simulink model "starmac_system"  (Simulink 7.1)
settings: Solver=ode5  StartTime=0.0  StopTime=30  FixedStep=.01  MaxStep=.01  RelTol=1e-4
undefined symbols (not defined in the file): ToverTh
libraries: xpcutilitieslib x19, simulink x10, xpclib x5, aero_sim_lib x1
settings Model: Creator=Administrator  LastModifiedBy=jporter  BufferReuse=off
settings OptimizationCC: BlockReduction=off  OptimizeBlockIOStorage=off  BufferReuse=off  ExpressionFolding=off  LocalBlockOutputs=off
settings HardwareCC: ProdIntDivRoundTo=Zero  ProdEndianess=LittleEndian  ProdHWDeviceType=Generic->32-bit x86 compatible
settings RTWCC: SystemTargetFile=xpctarget.tlc  TemplateMakefile=xpc_default_tmf  Description=xPC Target  ProcessScript=xpctarget_make_rtw_hook
settings xpcTargetCC: TargetFcnLib=ansi_tfl_table_tmw.mat  TargetFunctionLibrary=ANSI_C  CompOptLevelCompliant=off  PortableWordSizes=off  xPCisDownloadable=off

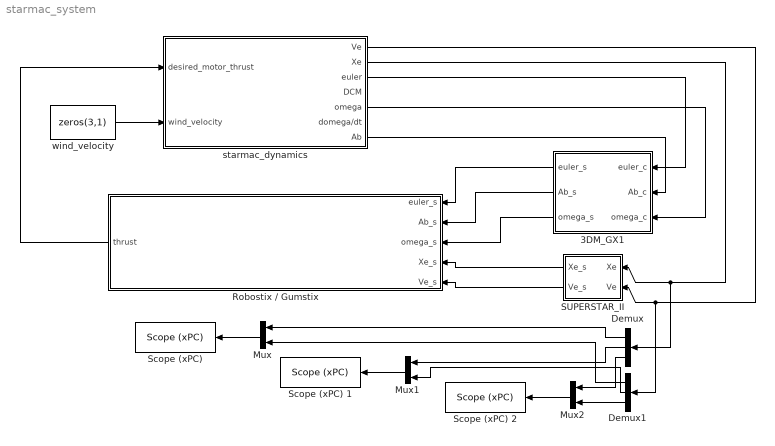
== system starmac_system ==
  3DM_GX1 : Subsystem  Orientation=left  mask{a_g_s=7000, g_max=5, g_g_s=8500, omega_max=300, Ts=.01}
      mask prompts: a_g_s "AccelGainScale:"; g_max "Max G (1 G = 9.81 m/s^2):"; g_g_s "GyroGainScale:"; omega_max "Mav Angular Velocity (deg/sec):"; Ts "Sample Rate (seconds):"
  Demux : Demux  Orientation=left  Outputs=3
  Demux1 : Demux  Orientation=left  Outputs=3
  Mux : Mux  Orientation=left  Inputs=2
  Mux1 : Mux  Orientation=left  Inputs=2
  Mux2 : Mux  Orientation=left  Inputs=2
  Robostix / Gumstix : Subsystem  Orientation=left
  SUPERSTAR_II : Subsystem  Orientation=left  mask{Ts=.2}
      mask prompts: Ts "Sample Rate (seconds):"
  "Scope (xPC) " : xpclib/Misc./Scope (xPC)   Orientation=left  SystemSampleTime=-1  scopeno=1  scopetype=Target  autostart=on  viewmode=Graphical redraw  formatstr='%15.6f'  grid=on  ylimits=[0,0]  nosamples=250  noprepostsamples=0  interleave=1  triggermode=FreeRun  triggersignal=1  triggerlevel=0.0  triggerslope=Either  triggerscope=1  triggersample=0  filename=data.dat  mode=Lazy  writesize=512  autorestart=off
  Scope (xPC) 1 : xpclib/Misc./Scope (xPC)   Orientation=left  SystemSampleTime=-1  scopeno=2  scopetype=Target  autostart=on  viewmode=Graphical redraw  formatstr='%15.6f'  grid=on  ylimits=[0,0]  nosamples=250  noprepostsamples=0  interleave=1  triggermode=FreeRun  triggersignal=1  triggerlevel=0.0  triggerslope=Either  triggerscope=1  triggersample=0  filename=data.dat  mode=Lazy  writesize=512  autorestart=off
  Scope (xPC) 2 : xpclib/Misc./Scope (xPC)   Orientation=left  SystemSampleTime=-1  scopeno=3  scopetype=Target  autostart=on  viewmode=Graphical redraw  formatstr='%15.6f'  grid=on  ylimits=[0,0]  nosamples=250  noprepostsamples=0  interleave=1  triggermode=FreeRun  triggersignal=1  triggerlevel=0.0  triggerslope=Either  triggerscope=1  triggersample=0  filename=data.dat  mode=Lazy  writesize=512  autorestart=off
  starmac_dynamics : Subsystem  AncestorBlock=aero_sim_lib/starmac_dynamics  mask{M=1.8263, tau_motor=0.1, b=0.1, select_sub=Select Subsystem}
      mask prompts: M "UAV Mass (kg) [M]:"; tau_motor "Motor Time constant (s)[tau_motor]:"; b "Viscus Drag Coef. (N-s/m)[b]:"; select_sub "Select a model Subsystem:"
      mask StyleString: edit,edit,edit,popup(Select Subsystem|M:starmac_motor_dynamics|B:starmac_blade_flapping_effects|6:6DOF_Euler_Angles)
      mask CallbackString:
      | |||gcb_d=gcb;
      | mask_str = get_param(gcb_d, 'MaskValues');
      | if strcmp(mask_str{4}(1),'M')
      |     open_system([gcb_d '/starmac_motor_dynamics'],'mask');
      | elseif strcmp(mask_str{4}(1),'B')
      |     open_system([gcb_d '/starmac_blade_flapping_effects'],'mask');
      | elseif strcmp(mask_str{4}(1),'6')
      |     open_system([gcb_d '/6DOF_Euler_Angles'],'mask');
      | else
      |     return
      | end
      | set_param(gcb_d,'select_sub','Select Subsystem');
  wind_velocity : Constant  Value=zeros(3,1)  OutDataType=sfix(16)  OutScaling=2^0
  wires:
  starmac_dynamics/3(euler) -> 3DM_GX1/1(euler_c)
  starmac_dynamics/7(Ab) -> 3DM_GX1/2(Ab_c)
  starmac_dynamics/5(omega) -> 3DM_GX1/3(omega_c)
  SUPERSTAR_II/1(Xe_s) -> Robostix / Gumstix/4(Xe_s)
  SUPERSTAR_II/2(Ve_s) -> Robostix / Gumstix/5(Ve_s)
  starmac_dynamics/2(Xe) -> SUPERSTAR_II/1(Xe), Demux/1
  starmac_dynamics/1(Ve) -> SUPERSTAR_II/2(Ve), Demux1/1
  wind_velocity/1 -> starmac_dynamics/2(wind_velocity)
  3DM_GX1/1(euler_s) -> Robostix / Gumstix/1(euler_s)
  3DM_GX1/2(Ab_s) -> Robostix / Gumstix/2(Ab_s)
  3DM_GX1/3(omega_s) -> Robostix / Gumstix/3(omega_s)
  Robostix / Gumstix/1(thrust) -> starmac_dynamics/1(desired_motor_thrust)
  Demux/1 -> Mux/1
  Demux/2 -> Mux1/1
  Demux/3 -> Mux2/1
  Demux1/1 -> Mux/2
  Demux1/2 -> Mux1/2
  Demux1/3 -> Mux2/2
  Mux/1 -> "Scope (xPC) "/1
  Mux1/1 -> Scope (xPC) 1/1
  Mux2/1 -> Scope (xPC) 2/1

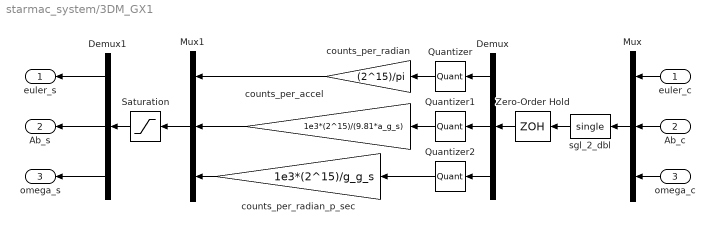
== system starmac_system/3DM_GX1 ==
  euler_c : Inport  Orientation=left
  Ab_c : Inport  Orientation=left  Port=2
  omega_c : Inport  Orientation=left  Port=3
  Demux : Demux  Orientation=left  Outputs=[3 3 3]
  Demux1 : Demux  Orientation=left  Outputs=[3 3 3]
  Mux : Mux  Orientation=left  Inputs=[3 3 3]
  Mux1 : Mux  Orientation=left  Inputs=3
  Quantizer : Quantizer  Orientation=left  QuantizationInterval=pi/(2^15)*ones(3,1)
  Quantizer1 : Quantizer  Orientation=left  QuantizationInterval=g_max*9.81/(2^15)*ones(3,1)
  Quantizer2 : Quantizer  Orientation=left  QuantizationInterval=(pi*omega_max/180)/(2^15)*ones(3,1)
  Saturation : Saturate  Orientation=left  UpperLimit=((2^15)-1)*ones(3*3,1)  LowerLimit=-(2^15)*ones(3*3,1)  OutDataType=sfix(16)  OutScaling=2^0
  Zero-Order Hold : ZeroOrderHold  Orientation=left  SampleTime=Ts
  counts_per_accel : Gain  Orientation=left  Gain=1e3*(2^15)/(9.81*a_g_s)  ParameterDataType=sfix(16)  ParameterScaling=2^0  OutDataType=sfix(16)  OutScaling=2^0
  counts_per_radian : Gain  Orientation=left  Gain=(2^15)/pi  ParameterDataType=sfix(16)  ParameterScaling=2^0  OutDataType=sfix(16)  OutScaling=2^0
  counts_per_radian_p_sec : Gain  Orientation=left  Gain=1e3*(2^15)/g_g_s  ParameterDataType=sfix(16)  ParameterScaling=2^0  OutDataType=sfix(16)  OutScaling=2^0
  sgl_2_dbl : DataTypeConversion  Orientation=left  OutDataTypeMode=single  OutDataType=sfix(16)  OutScaling=2^0  OutDataTypeStr=single
  euler_s : Outport  Orientation=left
  Ab_s : Outport  Orientation=left  Port=2
  omega_s : Outport  Orientation=left  Port=3
  wires:
  Mux/1 -> sgl_2_dbl/1
  euler_c/1 -> Mux/1
  Ab_c/1 -> Mux/2
  omega_c/1 -> Mux/3
  Zero-Order Hold/1 -> Demux/1
  Demux/1 -> Quantizer/1
  Demux/2 -> Quantizer1/1
  Quantizer/1 -> counts_per_radian/1
  Quantizer1/1 -> counts_per_accel/1
  counts_per_accel/1 -> Mux1/2
  counts_per_radian/1 -> Mux1/1
  Demux/3 -> Quantizer2/1
  counts_per_radian_p_sec/1 -> Mux1/3
  Quantizer2/1 -> counts_per_radian_p_sec/1
  Mux1/1 -> Saturation/1
  Saturation/1 -> Demux1/1
  Demux1/1 -> euler_s/1
  Demux1/2 -> Ab_s/1
  Demux1/3 -> omega_s/1
  sgl_2_dbl/1 -> Zero-Order Hold/1

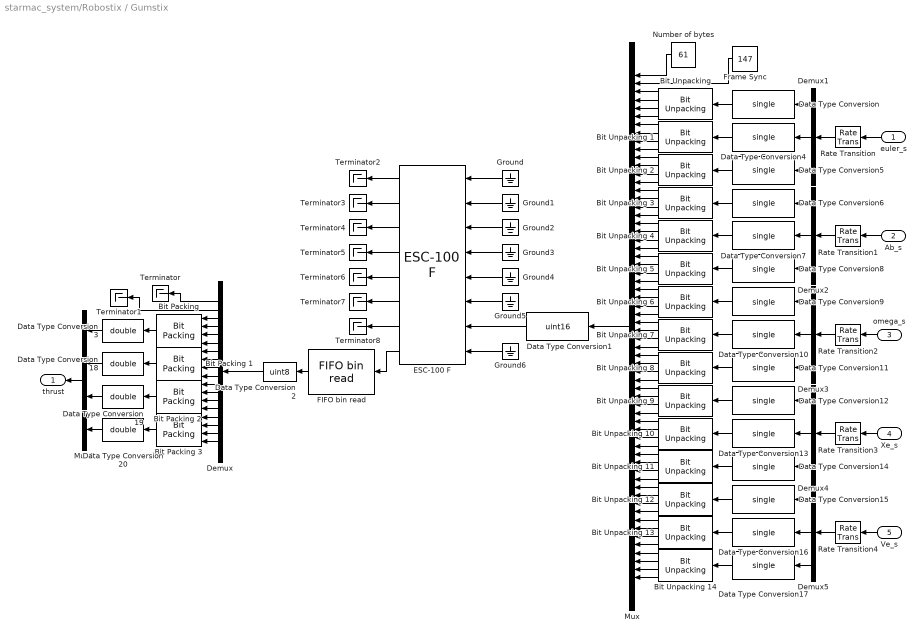
== system starmac_system/Robostix / Gumstix ==
  euler_s : Inport  Orientation=left
  Ab_s : Inport  Orientation=left  Port=2
  omega_s : Inport  Orientation=left  Port=3
  Xe_s : Inport  Orientation=left  Port=4
  Ve_s : Inport  Orientation=left  Port=5
  Bit Packing {,1..3} (4 alike) : xpcutilitieslib/Bit Packing   Orientation=left  MaskBitPatterns={[0:7], [8:15], [16:23], [24:31]}  MaskPackDataType=single  MaskPackDataSize=[1]
  Bit Unpacking {,1..14} (15 alike) : xpcutilitieslib/Bit Unpacking   Orientation=left  SignExtend=off  MaskBitPatterns={[0:7], [8:15], [16:23], [24:31]}  MaskPackDataType=single  MaskPackDataSize=[1]  MaskUnpackDataTypes={'uint8', 'uint8', 'uint8', 'uint8'}  MaskUnpackDataSizes={[1], [1], [1], [1]}
  Data Type Conversion{,4..17} (15 alike) : DataTypeConversion  Orientation=left  OutDataTypeMode=single  OutDataType=sfix(16)  OutScaling=2^0  OutDataTypeStr=single
  Data Type Conversion1 : DataTypeConversion  Orientation=left  OutDataTypeMode=uint16  OutDataType=sfix(16)  OutScaling=2^0  OutDataTypeStr=uint16  ConvertRealWorld=Stored Integer (SI)
  Data Type Conversion{3,18..20} (4 alike) : DataTypeConversion  Orientation=left  OutDataTypeMode=double  OutDataType=sfix(16)  OutScaling=2^0  OutDataTypeStr=double
  Data Type Conversion2 : DataTypeConversion  Orientation=left  OutDataTypeMode=uint8  OutDataType=sfix(16)  OutScaling=2^0  OutDataTypeStr=uint8
  Demux : Demux  Orientation=left  Outputs=18
  Demux{1..5} (5 alike) : Demux  Orientation=left  Outputs=3
  ESC-100 F : xpclib/RS232/Quatech/ESC-100/ESC-100 F  Orientation=left  SystemSampleTime=-1  group=Basic Setup  port=1  irqnum=10  slot=-1  baud1=57600  parity1=None  ndata1=8  nstop1=1  fifomode1=64 deep  rlevel1=half full  automode1=off  xmtfifosize1=1024  xmtdatatype1=count+16 bit uint  rcvfifosize1=1024  baud2=57600  parity2=None  ndata2=8  nstop2=1  fifomode2=64 deep  rlevel2=half full  automode2=off  xmtfifosize2=1024  xmtdatatype2=count+16 bit uint  rcvfifosize2=1024  baud3=57600  parity3=None  ndata3=8  nstop3=1  fifomode3=64 deep  rlevel3=half full  automode3=off  xmtfifosize3=1024  xmtdatatype3=count+16 bit uint  rcvfifosize3=1024  buad4=57600  parity4=None  ndata4=8  nstop4=1  fifomode4=64 deep  rlevel4=half full  automode4=off  xmtfifosize4=1024  xmtdatatype4=count+16 bit uint  rcvfifosize4=1024  baud5=57600  parity5=None  ndata5=8  nstop5=1  fifomode5=64 deep  rlevel5=half full  automode5=off  xmtfifosize5=1024  xmtdatatype5=count+16 bit uint  rcvfifosize5=1024  baud6=57600  parity6=None  ndata6=8  nstop6=1  fifomode6=64 deep  rlevel6=half full  automode6=off  xmtfifosize6=1024  xmtdatatype6=count+16 bit uint  rcvfifosize6=1024  baud7=57600  parity7=None  ndata7=8  nstop7=1  fifomode7=64 deep  rlevel7=half full  automode7=off  xmtfifosize7=1024  xmtdatatype7=count+16 bit uint  rcvfifosize7=1024  baud8=57600  parity8=None  ndata8=8  nstop8=1  fifomode8=64 deep  rlevel8=half full  automode8=off  xmtfifosize8=1024  xmtdatatype8=count+16 bit uint  rcvfifosize8=1024
  FIFO bin read : xpclib/RS232/FIFO bin read   Orientation=left  header={char([147])}  lengths=[17]  hold=Zero output if no new data  enable=off  maxsize=17  outputtype=count+16 bit uint  sampletime=-1
  Frame Sync : Constant  Orientation=left  Value=147  OutDataTypeMode=uint8  OutDataType=sfix(16)  OutScaling=2^0  OutDataTypeStr=uint8
  Ground{,1..6} (7 alike) : Ground  Orientation=left
  Mux : Mux  Orientation=left  Inputs=62
  Mux1 : Mux  Orientation=left
  Number of bytes : Constant  Orientation=left  Value=61  OutDataTypeMode=uint8  OutDataType=sfix(16)  OutScaling=2^0  OutDataTypeStr=uint8
  Rate Transition{,1..4} (5 alike) : RateTransition  Orientation=left
  Terminator{,1..8} (9 alike) : Terminator
  thrust : Outport  Orientation=left
  wires:
  Data Type Conversion/1 -> "Bit Unpacking "/1
  "Bit Unpacking "/4 -> Mux/6
  "Bit Unpacking "/3 -> Mux/5
  "Bit Unpacking "/2 -> Mux/4
  "Bit Unpacking "/1 -> Mux/3
  Frame Sync/1 -> Mux/2
  Number of bytes/1 -> Mux/1
  Mux/1 -> Data Type Conversion1/1
  Data Type Conversion1/1 -> ESC-100 F/7
  FIFO bin read/1 -> Data Type Conversion2/1
  Demux/1 -> Terminator/1
  Demux/2 -> Terminator1/1
  Demux/3 -> "Bit Packing "/1
  Demux/4 -> "Bit Packing "/2
  Demux/5 -> "Bit Packing "/3
  Demux/6 -> "Bit Packing "/4
  "Bit Packing "/1 -> Data Type Conversion3/1
  ESC-100 F/1 -> Terminator2/1
  ESC-100 F/2 -> Terminator3/1
  ESC-100 F/3 -> Terminator4/1
  ESC-100 F/4 -> Terminator5/1
  ESC-100 F/5 -> Terminator6/1
  ESC-100 F/6 -> Terminator7/1
  ESC-100 F/7 -> Terminator8/1
  Ground/1 -> ESC-100 F/1
  Ground1/1 -> ESC-100 F/2
  Ground2/1 -> ESC-100 F/3
  Ground3/1 -> ESC-100 F/4
  Ground4/1 -> ESC-100 F/5
  Ground5/1 -> ESC-100 F/6
  Ground6/1 -> ESC-100 F/8
  ESC-100 F/8 -> FIFO bin read/1
  Data Type Conversion2/1 -> Demux/1
  Data Type Conversion4/1 -> Bit Unpacking 1/1
  Bit Unpacking 1/4 -> Mux/10
  Bit Unpacking 1/3 -> Mux/9
  Bit Unpacking 1/2 -> Mux/8
  Bit Unpacking 1/1 -> Mux/7
  Data Type Conversion5/1 -> Bit Unpacking 2/1
  Bit Unpacking 2/4 -> Mux/14
  Bit Unpacking 2/3 -> Mux/13
  Bit Unpacking 2/2 -> Mux/12
  Bit Unpacking 2/1 -> Mux/11
  Data Type Conversion6/1 -> Bit Unpacking 3/1
  Bit Unpacking 3/4 -> Mux/18
  Bit Unpacking 3/3 -> Mux/17
  Bit Unpacking 3/2 -> Mux/16
  Bit Unpacking 3/1 -> Mux/15
  Data Type Conversion7/1 -> Bit Unpacking 4/1
  Bit Unpacking 4/4 -> Mux/22
  Bit Unpacking 4/3 -> Mux/21
  Bit Unpacking 4/2 -> Mux/20
  Bit Unpacking 4/1 -> Mux/19
  Data Type Conversion8/1 -> Bit Unpacking 5/1
  Bit Unpacking 5/4 -> Mux/26
  Bit Unpacking 5/3 -> Mux/25
  Bit Unpacking 5/2 -> Mux/24
  Bit Unpacking 5/1 -> Mux/23
  Data Type Conversion9/1 -> Bit Unpacking 6/1
  Bit Unpacking 6/4 -> Mux/30
  Bit Unpacking 6/3 -> Mux/29
  Bit Unpacking 6/2 -> Mux/28
  Bit Unpacking 6/1 -> Mux/27
  Data Type Conversion10/1 -> Bit Unpacking 7/1
  Bit Unpacking 7/4 -> Mux/34
  Bit Unpacking 7/3 -> Mux/33
  Bit Unpacking 7/2 -> Mux/32
  Bit Unpacking 7/1 -> Mux/31
  Data Type Conversion11/1 -> Bit Unpacking 8/1
  Bit Unpacking 8/4 -> Mux/38
  Bit Unpacking 8/3 -> Mux/37
  Bit Unpacking 8/2 -> Mux/36
  Bit Unpacking 8/1 -> Mux/35
  Data Type Conversion12/1 -> Bit Unpacking 9/1
  Bit Unpacking 9/4 -> Mux/42
  Bit Unpacking 9/3 -> Mux/41
  Bit Unpacking 9/2 -> Mux/40
  Bit Unpacking 9/1 -> Mux/39
  Data Type Conversion13/1 -> Bit Unpacking 10/1
  Bit Unpacking 10/4 -> Mux/46
  Bit Unpacking 10/3 -> Mux/45
  Bit Unpacking 10/2 -> Mux/44
  Bit Unpacking 10/1 -> Mux/43
  Data Type Conversion14/1 -> Bit Unpacking 11/1
  Bit Unpacking 11/4 -> Mux/50
  Bit Unpacking 11/3 -> Mux/49
  Bit Unpacking 11/2 -> Mux/48
  Bit Unpacking 11/1 -> Mux/47
  Data Type Conversion15/1 -> Bit Unpacking 12/1
  Bit Unpacking 12/4 -> Mux/54
  Bit Unpacking 12/3 -> Mux/53
  Bit Unpacking 12/2 -> Mux/52
  Bit Unpacking 12/1 -> Mux/51
  Data Type Conversion16/1 -> Bit Unpacking 13/1
  Bit Unpacking 13/4 -> Mux/58
  Bit Unpacking 13/3 -> Mux/57
  Bit Unpacking 13/2 -> Mux/56
  Bit Unpacking 13/1 -> Mux/55
  Data Type Conversion17/1 -> Bit Unpacking 14/1
  Bit Unpacking 14/4 -> Mux/62
  Bit Unpacking 14/3 -> Mux/61
  Bit Unpacking 14/2 -> Mux/60
  Bit Unpacking 14/1 -> Mux/59
  Demux1/1 -> Data Type Conversion/1
  Demux1/2 -> Data Type Conversion4/1
  Demux1/3 -> Data Type Conversion5/1
  euler_s/1 -> Rate Transition/1
  Ab_s/1 -> Rate Transition1/1
  Demux2/1 -> Data Type Conversion6/1
  Demux2/2 -> Data Type Conversion7/1
  Demux2/3 -> Data Type Conversion8/1
  omega_s/1 -> Rate Transition2/1
  Demux3/1 -> Data Type Conversion9/1
  Demux3/2 -> Data Type Conversion10/1
  Demux3/3 -> Data Type Conversion11/1
  Xe_s/1 -> Rate Transition3/1
  Demux4/1 -> Data Type Conversion12/1
  Demux4/2 -> Data Type Conversion13/1
  Demux4/3 -> Data Type Conversion14/1
  Ve_s/1 -> Rate Transition4/1
  Demux5/1 -> Data Type Conversion15/1
  Demux5/2 -> Data Type Conversion16/1
  Demux5/3 -> Data Type Conversion17/1
  Demux/7 -> Bit Packing 1/1
  Demux/8 -> Bit Packing 1/2
  Demux/9 -> Bit Packing 1/3
  Demux/10 -> Bit Packing 1/4
  Bit Packing 1/1 -> Data Type Conversion18/1
  Demux/11 -> Bit Packing 2/1
  Demux/12 -> Bit Packing 2/2
  Demux/13 -> Bit Packing 2/3
  Demux/14 -> Bit Packing 2/4
  Bit Packing 2/1 -> Data Type Conversion19/1
  Demux/15 -> Bit Packing 3/1
  Demux/16 -> Bit Packing 3/2
  Demux/17 -> Bit Packing 3/3
  Demux/18 -> Bit Packing 3/4
  Bit Packing 3/1 -> Data Type Conversion20/1
  Data Type Conversion3/1 -> Mux1/1
  Data Type Conversion18/1 -> Mux1/2
  Data Type Conversion19/1 -> Mux1/3
  Data Type Conversion20/1 -> Mux1/4
  Mux1/1 -> thrust/1
  Rate Transition/1 -> Demux1/1
  Rate Transition1/1 -> Demux2/1
  Rate Transition2/1 -> Demux3/1
  Rate Transition3/1 -> Demux4/1
  Rate Transition4/1 -> Demux5/1

== system starmac_system/SUPERSTAR_II ==
  Xe : Inport  Orientation=left
  Ve : Inport  Orientation=left  Port=2
  Demux : Demux  Orientation=left  Outputs=[3 3]
  Mux : Mux  Orientation=left  Inputs=[3 3]
  ZOH : ZeroOrderHold  Orientation=left  SampleTime=Ts
  sgl_2_dbl : DataTypeConversion  Orientation=left  OutDataTypeMode=single  OutDataType=sfix(16)  OutScaling=2^0  OutDataTypeStr=single
  Xe_s : Outport  Orientation=left
  Ve_s : Outport  Orientation=left  Port=2
  wires:
  ZOH/1 -> Demux/1
  Ve/1 -> Mux/2
  Xe/1 -> Mux/1
  Mux/1 -> sgl_2_dbl/1
  Demux/1 -> Xe_s/1
  Demux/2 -> Ve_s/1
  sgl_2_dbl/1 -> ZOH/1

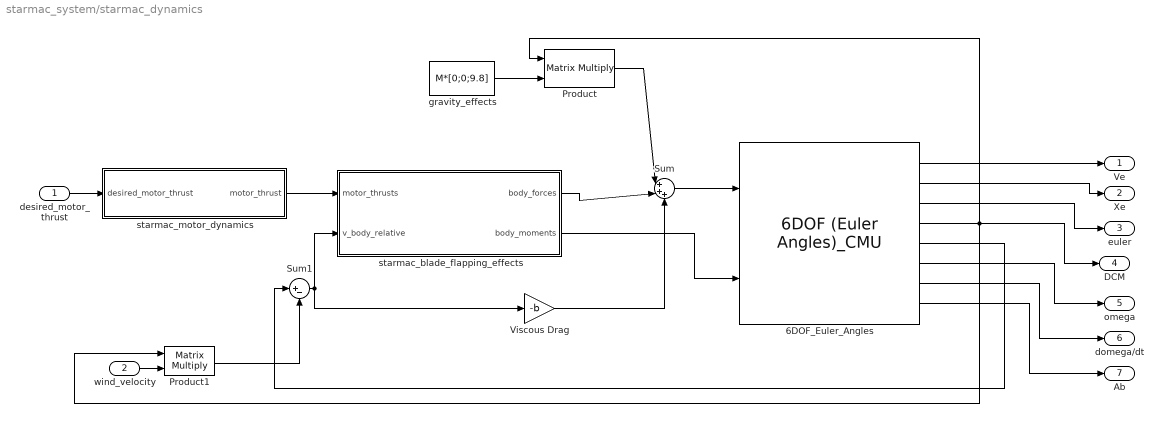
== system starmac_system/starmac_dynamics ==
  desired_motor_thrust : Inport  OutDataType=sfix(16)  OutScaling=2^0
  wind_velocity : Inport  Port=2  OutDataType=sfix(16)  OutScaling=2^0
  6DOF_Euler_Angles : aero_sim_lib/6DOF (Euler Angles)_CMU  SystemSampleTime=-1  XYZe_0=[0.1;0.2;0]  Vb_0=[0;0;0]  euler_0=[0;0;0]  omega_0=[0;0;0]  M=M  I=diag([0.02759 0.02771 0.04806])
  Product : Product  Multiplication=Matrix(*)  OutDataType=sfix(16)  OutScaling=2^0  RndMeth=Zero
  Product1 : Product  Multiplication=Matrix(*)  OutDataType=sfix(16)  OutScaling=2^0  RndMeth=Zero
  Sum : Sum  Inputs=|+++  OutDataType=sfix(16)  OutScaling=2^0
  Sum1 : Sum  Inputs=|+-  OutDataType=sfix(16)  OutScaling=2^0
  Viscous Drag : Gain  Gain=-b  ParameterDataType=sfix(16)  ParameterScaling=2^0  OutDataType=sfix(16)  OutScaling=2^0
  gravity_effects : Constant  Value=M*[0;0;9.8]  OutDataType=sfix(16)  OutScaling=2^0
  starmac_blade_flapping_effects : Subsystem  AncestorBlock=aero_sim_lib/starmac_blade_flapping_effects  mask{select_sub=Select Subsystem}
      mask prompts: select_sub "Select Subsystem:"
      mask help:
      | Allows user to set parameters of various subsystems
      | within the Blade Flapping Effects Model
      mask Help:
      | Select a Subsystem To Set Various
      | Sub System Parameters
      mask StyleString: popup(Select Subsystem|V:starmac_vertical_effect_dynamics|B:starmac_body_moments|F:starmac_flapping_dynamics)
      mask CallbackString:
      | gcb_c=gcb;
      | mask_str = get_param(gcb_c, 'MaskValues');
      | if strcmp(mask_str{1}(1),'V')
      |     open_system([gcb_c '/starmac_vertical_effect_dynamics'],'mask');
      | elseif strcmp(mask_str{1}(1),'B')
      |     open_system([gcb_c '/starmac_body_moments'],'mask');
      | elseif strcmp(mask_str{1}(1),'F')
      |     open_system([gcb_c '/starmac_flapping_dynamics'],'mask');
      | else
      |     return
      | end
      | set_param(gcb_c,'select_sub','Select Subsystem');
  starmac_motor_dynamics : Subsystem  AncestorBlock=aero_sim_lib/starmac_motor_dynamics  mask{tau_motor=tau_motor, T_nom=M*9.8/4, thrust_max=9.8, thrust_min=0, motor_lag_enable=on, motor_variance=(.05*9.8/4)^2, Ts=.01}
      mask prompts: tau_motor "tau_motor (seconds):"; T_nom "nominal thrust (N):"; thrust_max "maximum thrust (N):"; thrust_min "minimum thrust (N):"; motor_lag_enable "Motor Lag Enabled:"; motor_variance "Motor Variance [motor_variance]:"; Ts "Motor Update Rate (seconds):"
  Ve : Outport  OutDataType=sfix(16)  OutScaling=2^0
  Xe : Outport  Port=2  OutDataType=sfix(16)  OutScaling=2^0
  euler : Outport  Port=3  OutDataType=sfix(16)  OutScaling=2^0
  DCM : Outport  Port=4  OutDataType=sfix(16)  OutScaling=2^0
  omega : Outport  Port=5  OutDataType=sfix(16)  OutScaling=2^0
  domega/dt : Outport  Port=6  OutDataType=sfix(16)  OutScaling=2^0
  Ab : Outport  Port=7  OutDataType=sfix(16)  OutScaling=2^0
  wires:
  6DOF_Euler_Angles/8 -> Ab/1
  6DOF_Euler_Angles/7 -> domega/dt/1
  6DOF_Euler_Angles/6 -> omega/1
  6DOF_Euler_Angles/3 -> euler/1
  6DOF_Euler_Angles/2 -> Xe/1
  6DOF_Euler_Angles/1 -> Ve/1
  starmac_motor_dynamics/1(motor_thrust) -> starmac_blade_flapping_effects/1(motor_thrusts)
  Product/1 -> Sum/1
  Sum/1 -> 6DOF_Euler_Angles/1
  6DOF_Euler_Angles/4 -> DCM/1, Product/1, Product1/1
  gravity_effects/1 -> Product/2
  Sum1/1 -> starmac_blade_flapping_effects/2(v_body_relative), Viscous Drag/1
  Product1/1 -> Sum1/2
  6DOF_Euler_Angles/5 -> Sum1/1
  Viscous Drag/1 -> Sum/3
  starmac_blade_flapping_effects/2(body_moments) -> 6DOF_Euler_Angles/2
  starmac_blade_flapping_effects/1(body_forces) -> Sum/2
  desired_motor_thrust/1 -> starmac_motor_dynamics/1(desired_motor_thrust)
  wind_velocity/1 -> Product1/2

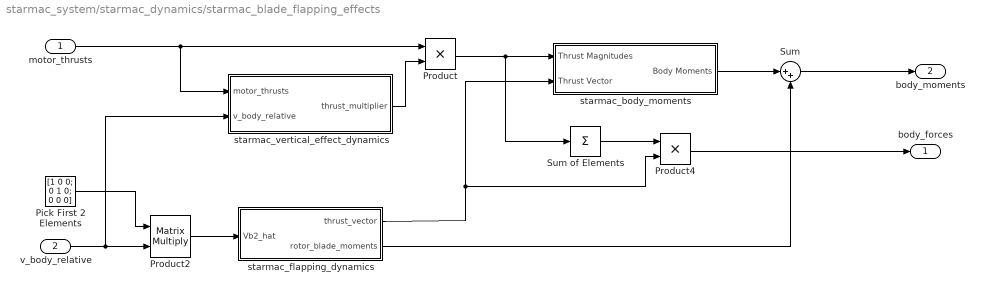
== system starmac_system/starmac_dynamics/starmac_blade_flapping_effects ==
  motor_thrusts : Inport  OutDataType=sfix(16)  OutScaling=2^0
  v_body_relative : Inport  Port=2  OutDataType=sfix(16)  OutScaling=2^0
  Pick First 2 Elements : Constant  Value=[1 0 0; 0 1 0; 0 0 0]  OutDataType=sfix(16)  OutScaling=2^0
  Product : Product  OutDataType=sfix(16)  OutScaling=2^0  RndMeth=Zero
  Product2 : Product  Multiplication=Matrix(*)  OutDataType=sfix(16)  OutScaling=2^0  RndMeth=Zero
  Product4 : Product  OutDataType=sfix(16)  OutScaling=2^0  RndMeth=Zero
  Sum : Sum  Inputs=|++  OutDataType=sfix(16)  OutScaling=2^0
  Sum of Elements : Sum  Inputs=+  OutDataType=sfix(16)  OutScaling=2^-10
  starmac_body_moments : Subsystem  AncestorBlock=aero_sim_lib/starmac_body_moments  mask{dx=.3048, dz=.07, K_torque=.47}
  starmac_flapping_dynamics : Subsystem  AncestorBlock=aero_sim_lib/starmac_flapping_dynamics  mask{K_a1s=.009, K_beta=.23}
  starmac_vertical_effect_dynamics : Subsystem  AncestorBlock=aero_sim_lib/starmac_vertical_effect_dynamics  mask{tau_motor=tau_motor, R=0.127, Alpha=(pi/180)*[-85:5:85], Vinf=[0:0.5:6], Thrust=9.8*[0.3:0.02:0.8]}
      mask prompts: tau_motor "motor time constant (s)"; R "radius of propeller (m)"; Alpha "Alpha (radians)"; Vinf "Vinf (radians)"; Thrust "Propeller Thrust (N)"
      mask init:
      | rho = 1.2;
      | A = pi*R^2;
      | Vh = sqrt(Thrust/(2*rho*A));
      | for i = 1:length(Vh)
      |     for j = 1:length(Vinf)
      |         for k = 1:length(Alpha)
      |             Vi(k,j,i) = find_vi(Vh(i),Vinf(j),Alpha(k));
      |             ToverTh(k,j,i) = min(10,max(0.1,Vh(i)/(Vi(k,j,i)+Vinf(j)*sin(Alpha(k)))));
      |         end
      |     end
      | end
  body_forces : Outport  OutDataType=sfix(16)  OutScaling=2^0
  body_moments : Outport  Port=2  OutDataType=sfix(16)  OutScaling=2^0
  wires:
  starmac_flapping_dynamics/2(rotor_blade_moments) -> Sum/2
  Sum/1 -> body_moments/1
  starmac_body_moments/1(Body Moments) -> Sum/1
  starmac_flapping_dynamics/1(thrust_vector) -> Product4/2, starmac_body_moments/2(Thrust Vector)
  Product4/1 -> body_forces/1
  Sum of Elements/1 -> Product4/1
  Product2/1 -> starmac_flapping_dynamics/1(Vb2_hat)
  v_body_relative/1 -> Product2/2, starmac_vertical_effect_dynamics/2(v_body_relative)
  Pick First 2 Elements/1 -> Product2/1
  motor_thrusts/1 -> Product/1, starmac_vertical_effect_dynamics/1(motor_thrusts)
  starmac_vertical_effect_dynamics/1(thrust_multiplier) -> Product/2
  Product/1 -> Sum of Elements/1, starmac_body_moments/1(Thrust Magnitudes)

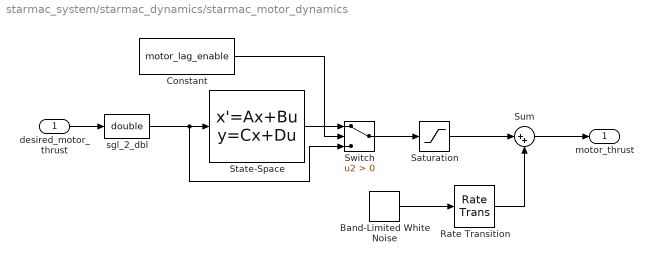
== system starmac_system/starmac_dynamics/starmac_motor_dynamics ==
  desired_motor_thrust : Inport  OutDataType=sfix(16)  OutScaling=2^0
  Band-Limited White Noise : simulink/Sources/Band-Limited White Noise  SystemSampleTime=-1  Cov=Ts*motor_variance*ones(4,1)  Ts=Ts  seed=22341+[0 1 2 3]'
  Constant : Constant  Value=motor_lag_enable  OutDataType=sfix(16)  OutScaling=2^0
  Rate Transition : RateTransition
  Saturation : Saturate  UpperLimit=thrust_max*ones(4,1)  LowerLimit=thrust_min*ones(4,1)
  State-Space : StateSpace  A=-(1/tau_motor)*eye(4)  B=(1/tau_motor)*eye(4)  C=eye(4)  D=zeros(4,4)  X0=T_nom*ones(4,1)
  Sum : Sum  Inputs=|++  OutDataType=sfix(16)  OutScaling=2^0
  Switch : Switch  Criteria=u2 > Threshold  OutDataType=sfix(16)  OutScaling=2^0
  sgl_2_dbl : DataTypeConversion  OutDataTypeMode=double  OutDataType=sfix(16)  OutScaling=2^0  OutDataTypeStr=double
  motor_thrust : Outport  OutDataType=sfix(16)  OutScaling=2^0
  wires:
  desired_motor_thrust/1 -> sgl_2_dbl/1
  Sum/1 -> motor_thrust/1
  Saturation/1 -> Sum/1
  Band-Limited White Noise/1 -> Rate Transition/1
  State-Space/1 -> Switch/1
  Switch/1 -> Saturation/1
  Constant/1 -> Switch/2
  Rate Transition/1 -> Sum/2
  sgl_2_dbl/1 -> Switch/3, State-Space/1

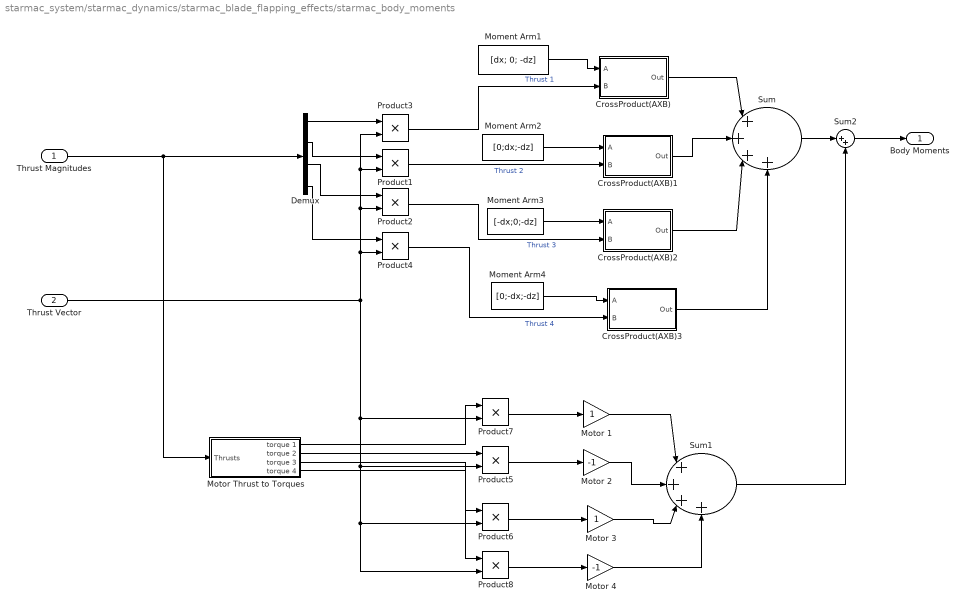
== system starmac_system/starmac_dynamics/starmac_blade_flapping_effects/starmac_body_moments ==
  Thrust Magnitudes : Inport  OutDataType=sfix(16)  OutScaling=2^0
  Thrust Vector : Inport  Port=2  OutDataType=sfix(16)  OutScaling=2^0
  CrossProduct(AXB) : Subsystem
  CrossProduct(AXB)1 : Subsystem
  CrossProduct(AXB)2 : Subsystem
  CrossProduct(AXB)3 : Subsystem
  Demux : Demux
  Moment Arm1 : Constant  Value=[dx; 0; -dz]  OutDataType=sfix(16)  OutScaling=2^0
  Moment Arm2 : Constant  Value=[0;dx;-dz]  OutDataType=sfix(16)  OutScaling=2^0
  Moment Arm3 : Constant  Value=[-dx;0;-dz]  OutDataType=sfix(16)  OutScaling=2^0
  Moment Arm4 : Constant  Value=[0;-dx;-dz]  OutDataType=sfix(16)  OutScaling=2^0
  Motor 1 : Gain  ParameterDataType=sfix(16)  ParameterScaling=2^0  OutDataType=sfix(16)  OutScaling=2^0
  Motor 2 : Gain  Gain=-1  ParameterDataType=sfix(16)  ParameterScaling=2^0  OutDataType=sfix(16)  OutScaling=2^0
  Motor 3 : Gain  ParameterDataType=sfix(16)  ParameterScaling=2^0  OutDataType=sfix(16)  OutScaling=2^0
  Motor 4 : Gain  Gain=-1  ParameterDataType=sfix(16)  ParameterScaling=2^0  OutDataType=sfix(16)  OutScaling=2^0
  Motor Thrust to Torques : Subsystem
  Product{1..8} (8 alike) : Product  OutDataType=sfix(16)  OutScaling=2^0  RndMeth=Zero
  Sum : Sum  Inputs=|++++  OutDataType=sfix(16)  OutScaling=2^0
  Sum1 : Sum  Inputs=|++++  OutDataType=sfix(16)  OutScaling=2^0
  Sum2 : Sum  Inputs=|++  OutDataType=sfix(16)  OutScaling=2^0
  Body Moments : Outport  OutDataType=sfix(16)  OutScaling=2^0
  wires:
  CrossProduct(AXB)1/1(Out) -> Sum/2
  Motor Thrust to Torques/4(torque 4) -> Product8/1
  Motor Thrust to Torques/3(torque 3) -> Product6/1
  Motor Thrust to Torques/2(torque 2) -> Product5/1
  Motor Thrust to Torques/1(torque 1) -> Product7/1
  Product8/1 -> Motor 4/1
  Product6/1 -> Motor 3/1
  Product5/1 -> Motor 2/1
  Product7/1 -> Motor 1/1
  Sum2/1 -> Body Moments/1
  Sum1/1 -> Sum2/2
  Sum/1 -> Sum2/1
  Motor 4/1 -> Sum1/4
  Motor 3/1 -> Sum1/3
  Motor 2/1 -> Sum1/2
  Motor 1/1 -> Sum1/1
  CrossProduct(AXB)3/1(Out) -> Sum/4
  CrossProduct(AXB)2/1(Out) -> Sum/3
  CrossProduct(AXB)/1(Out) -> Sum/1
  Product4/1 -> CrossProduct(AXB)3/2(B)  "Thrust 4"
  Moment Arm4/1 -> CrossProduct(AXB)3/1(A)
  Product2/1 -> CrossProduct(AXB)2/2(B)  "Thrust 3"
  Moment Arm3/1 -> CrossProduct(AXB)2/1(A)
  Product1/1 -> CrossProduct(AXB)1/2(B)  "Thrust 2"
  Moment Arm2/1 -> CrossProduct(AXB)1/1(A)
  Product3/1 -> CrossProduct(AXB)/2(B)  "Thrust 1"
  Moment Arm1/1 -> CrossProduct(AXB)/1(A)
  Thrust Vector/1 -> Product8/2, Product6/2, Product5/2, Product7/2, Product4/2, Product2/2, Product1/2, Product3/2
  Demux/4 -> Product4/1
  Demux/3 -> Product2/1
  Demux/2 -> Product1/1
  Demux/1 -> Product3/1
  Thrust Magnitudes/1 -> Motor Thrust to Torques/1(Thrusts), Demux/1

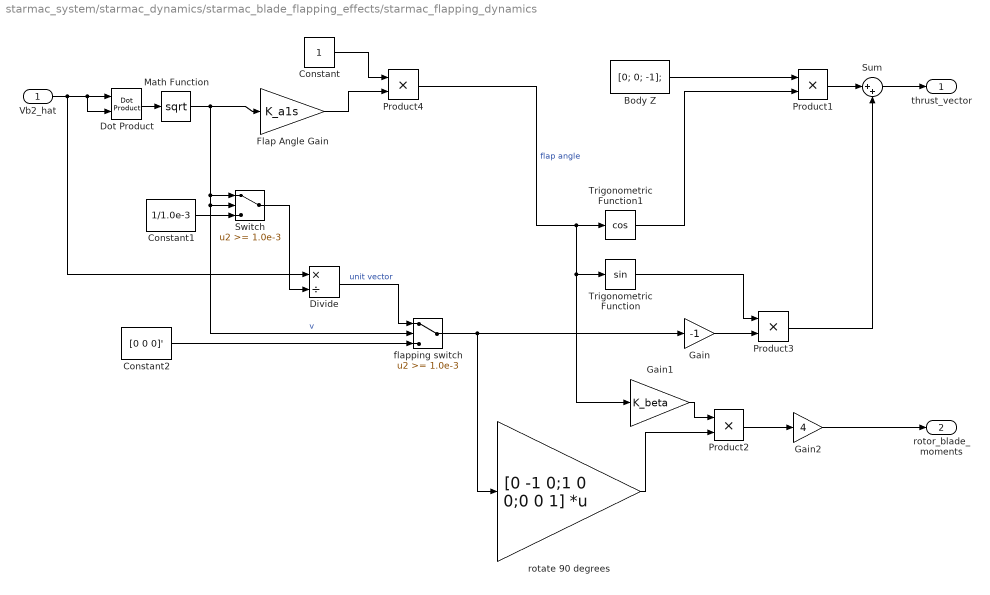
== system starmac_system/starmac_dynamics/starmac_blade_flapping_effects/starmac_flapping_dynamics ==
  Vb2_hat : Inport  OutDataType=sfix(16)  OutScaling=2^0
  "Body Z " : Constant  Value=[0; 0; -1];  OutDataType=sfix(16)  OutScaling=2^0
  Constant : Constant  OutDataType=sfix(16)  OutScaling=2^0
  Constant1 : Constant  Value=1/1.0e-3  OutDataType=sfix(16)  OutScaling=2^0
  Constant2 : Constant  Value=[0 0 0]'  OutDataType=sfix(16)  OutScaling=2^0
  Divide : Product  Inputs=*/  OutDataType=sfix(16)  OutScaling=2^-10
  Dot Product : simulink/Math Operations/Dot Product  InputSameDT=on  OutDataType=sfix(16)  OutScaling=2^-10  DoSatur=off
  Flap Angle Gain : Gain  Gain=K_a1s  ParameterDataType=sfix(16)  ParameterScaling=2^0  OutDataType=sfix(16)  OutScaling=2^0
  Gain : Gain  Gain=-1  ParameterDataType=sfix(16)  ParameterScaling=2^0  OutDataType=sfix(16)  OutScaling=2^0
  Gain1 : Gain  Gain=K_beta  ParameterDataType=sfix(16)  ParameterScaling=2^0  OutDataType=sfix(16)  OutScaling=2^0
  Gain2 : Gain  Gain=4  ParameterDataType=sfix(16)  ParameterScaling=2^0  OutDataType=sfix(16)  OutScaling=2^0
  Math Function : Math  Operator=sqrt  OutDataType=sfix(16)  OutScaling=2^0  SaturateOnIntegerOverflow=on
  Product{1..4} (4 alike) : Product  OutDataType=sfix(16)  OutScaling=2^0  RndMeth=Zero
  Sum : Sum  Inputs=|++  OutDataType=sfix(16)  OutScaling=2^0
  Switch : Switch  Threshold=1.0e-3
  Trigonometric Function : Trigonometry
  Trigonometric Function1 : Trigonometry  Operator=cos
  flapping switch : Switch  Threshold=1.0e-3
  rotate 90 degrees : Gain  Gain=[0 -1 0;1 0 0;0 0 1]  Multiplication=Matrix(K*u)  ParameterDataType=sfix(16)  ParameterScaling=2^0  OutDataType=sfix(16)  OutScaling=2^0
  thrust_vector : Outport  OutDataType=sfix(16)  OutScaling=2^0
  rotor_blade_moments : Outport  Port=2  OutDataType=sfix(16)  OutScaling=2^0
  wires:
  Constant/1 -> Product4/1
  Flap Angle Gain/1 -> Product4/2
  Gain1/1 -> Product2/1
  rotate 90 degrees/1 -> Product2/2
  Product2/1 -> Gain2/1
  Constant2/1 -> flapping switch/3
  flapping switch/1 -> rotate 90 degrees/1, Gain/1
  Divide/1 -> flapping switch/1  "unit vector"
  Constant1/1 -> Switch/3
  Switch/1 -> Divide/2
  Gain2/1 -> rotor_blade_moments/1
  Sum/1 -> thrust_vector/1
  "Body Z "/1 -> Product1/1
  Product1/1 -> Sum/1
  Gain/1 -> Product3/2
  Product3/1 -> Sum/2
  Trigonometric Function/1 -> Product3/1
  Trigonometric Function1/1 -> Product1/2
  Math Function/1 -> Flap Angle Gain/1, flapping switch/2, Switch/2, Switch/1  "v"
  Dot Product/1 -> Math Function/1
  Vb2_hat/1 -> Divide/1, Dot Product/2, Dot Product/1
  Product4/1 -> Gain1/1, Trigonometric Function/1, Trigonometric Function1/1  "flap angle"

== system starmac_system/starmac_dynamics/starmac_blade_flapping_effects/starmac_vertical_effect_dynamics ==
  motor_thrusts : Inport  OutDataType=sfix(16)  OutScaling=2^0
  v_body_relative : Inport  Port=2  OutDataType=sfix(16)  OutScaling=2^0
  Demux : Demux
  Mux : Mux
  starmac_motor_vertical_effect_dynamics : Subsystem  AncestorBlock=aero_sim_lib/starmac_motor_vertical_effect_dynamics  mask{tau_motor=tau_motor, R=R, Alpha=Alpha, Vinf=Vinf, Vh=Vh, ToverTh=ToverTh}
      mask prompts: tau_motor "motor time constant (s)"; R "radius of propeller (m)"; Alpha "Alpha (radians):"; Vinf "Vinf (m/s):"; Vh "Vh (m/s):"
      mask init:
      | rho=1.2;    % kg/m^3, density of air
      | A = pi*R^2; % m^2, area swept out by 1 rotor
  starmac_motor_vertical_effect_dynamics1 : Subsystem  AncestorBlock=aero_sim_lib/starmac_motor_vertical_effect_dynamics  mask{tau_motor=tau_motor, R=R, Alpha=Alpha, Vinf=Vinf, Vh=Vh, ToverTh=ToverTh}
      mask prompts: tau_motor "motor time constant (s)"; R "radius of propeller (m)"; Alpha "Alpha (radians):"; Vinf "Vinf (m/s):"; Vh "Vh (m/s):"
      mask init:
      | rho=1.2;    % kg/m^3, density of air
      | A = pi*R^2; % m^2, area swept out by 1 rotor
  starmac_motor_vertical_effect_dynamics2 : Subsystem  AncestorBlock=aero_sim_lib/starmac_motor_vertical_effect_dynamics  mask{tau_motor=tau_motor, R=R, Alpha=Alpha, Vinf=Vinf, Vh=Vh, ToverTh=ToverTh}
      mask prompts: tau_motor "motor time constant (s)"; R "radius of propeller (m)"; Alpha "Alpha (radians):"; Vinf "Vinf (m/s):"; Vh "Vh (m/s):"
      mask init:
      | rho=1.2;    % kg/m^3, density of air
      | A = pi*R^2; % m^2, area swept out by 1 rotor
  starmac_motor_vertical_effect_dynamics3 : Subsystem  AncestorBlock=aero_sim_lib/starmac_motor_vertical_effect_dynamics  mask{tau_motor=tau_motor, R=R, Alpha=Alpha, Vinf=Vinf, Vh=Vh, ToverTh=ToverTh}
      mask prompts: tau_motor "motor time constant (s)"; R "radius of propeller (m)"; Alpha "Alpha (radians):"; Vinf "Vinf (m/s):"; Vh "Vh (m/s):"
      mask init:
      | rho=1.2;    % kg/m^3, density of air
      | A = pi*R^2; % m^2, area swept out by 1 rotor
  thrust_multiplier : Outport  OutDataType=sfix(16)  OutScaling=2^0
  wires:
  motor_thrusts/1 -> Demux/1
  Mux/1 -> thrust_multiplier/1
  Demux/1 -> starmac_motor_vertical_effect_dynamics/1(motor_thrusts)
  Demux/2 -> starmac_motor_vertical_effect_dynamics1/1(motor_thrusts)
  Demux/3 -> starmac_motor_vertical_effect_dynamics2/1(motor_thrusts)
  Demux/4 -> starmac_motor_vertical_effect_dynamics3/1(motor_thrusts)
  starmac_motor_vertical_effect_dynamics/1(thrust_multiplier) -> Mux/1
  starmac_motor_vertical_effect_dynamics1/1(thrust_multiplier) -> Mux/2
  starmac_motor_vertical_effect_dynamics2/1(thrust_multiplier) -> Mux/3
  starmac_motor_vertical_effect_dynamics3/1(thrust_multiplier) -> Mux/4
  v_body_relative/1 -> starmac_motor_vertical_effect_dynamics2/2(v_body_relative), starmac_motor_vertical_effect_dynamics3/2(v_body_relative), starmac_motor_vertical_effect_dynamics1/2(v_body_relative), starmac_motor_vertical_effect_dynamics/2(v_body_relative)

== system starmac_system/starmac_dynamics/starmac_blade_flapping_effects/starmac_body_moments/CrossProduct(AXB) ==
  A : Inport  OutDataType=sfix(16)  OutScaling=2^0
  B : Inport  Port=2  OutDataType=sfix(16)  OutScaling=2^0
  Fcn : Fcn  Expr=u[2]*u[6]-u[3]*u[5]
  Fcn1 : Fcn  Expr=u[3]*u[4]-u[1]*u[6]
  Fcn2 : Fcn  Expr=u[1]*u[5]-u[2]*u[4]
  Mux : Mux  Inputs=2
  Mux1 : Mux  Inputs=3
  Out : Outport  OutDataType=sfix(16)  OutScaling=2^0
  wires:
  Mux1/1 -> Out/1
  Fcn2/1 -> Mux1/3
  Fcn1/1 -> Mux1/2
  Fcn/1 -> Mux1/1
  Mux/1 -> Fcn2/1, Fcn1/1, Fcn/1
  B/1 -> Mux/2
  A/1 -> Mux/1

== system starmac_system/starmac_dynamics/starmac_blade_flapping_effects/starmac_body_moments/CrossProduct(AXB)1 ==
  A : Inport  OutDataType=sfix(16)  OutScaling=2^0
  B : Inport  Port=2  OutDataType=sfix(16)  OutScaling=2^0
  Fcn : Fcn  Expr=u[2]*u[6]-u[3]*u[5]
  Fcn1 : Fcn  Expr=u[3]*u[4]-u[1]*u[6]
  Fcn2 : Fcn  Expr=u[1]*u[5]-u[2]*u[4]
  Mux : Mux  Inputs=2
  Mux1 : Mux  Inputs=3
  Out : Outport  OutDataType=sfix(16)  OutScaling=2^0
  wires:
  A/1 -> Mux/1
  B/1 -> Mux/2
  Mux/1 -> Fcn/1, Fcn1/1, Fcn2/1
  Fcn/1 -> Mux1/1
  Fcn1/1 -> Mux1/2
  Fcn2/1 -> Mux1/3
  Mux1/1 -> Out/1

== system starmac_system/starmac_dynamics/starmac_blade_flapping_effects/starmac_body_moments/CrossProduct(AXB)2 ==
  A : Inport  OutDataType=sfix(16)  OutScaling=2^0
  B : Inport  Port=2  OutDataType=sfix(16)  OutScaling=2^0
  Fcn : Fcn  Expr=u[2]*u[6]-u[3]*u[5]
  Fcn1 : Fcn  Expr=u[3]*u[4]-u[1]*u[6]
  Fcn2 : Fcn  Expr=u[1]*u[5]-u[2]*u[4]
  Mux : Mux  Inputs=2
  Mux1 : Mux  Inputs=3
  Out : Outport  OutDataType=sfix(16)  OutScaling=2^0
  wires:
  Mux1/1 -> Out/1
  Fcn2/1 -> Mux1/3
  Fcn1/1 -> Mux1/2
  Fcn/1 -> Mux1/1
  Mux/1 -> Fcn2/1, Fcn1/1, Fcn/1
  B/1 -> Mux/2
  A/1 -> Mux/1

== system starmac_system/starmac_dynamics/starmac_blade_flapping_effects/starmac_body_moments/CrossProduct(AXB)3 ==
  A : Inport  OutDataType=sfix(16)  OutScaling=2^0
  B : Inport  Port=2  OutDataType=sfix(16)  OutScaling=2^0
  Fcn : Fcn  Expr=u[2]*u[6]-u[3]*u[5]
  Fcn1 : Fcn  Expr=u[3]*u[4]-u[1]*u[6]
  Fcn2 : Fcn  Expr=u[1]*u[5]-u[2]*u[4]
  Mux : Mux  Inputs=2
  Mux1 : Mux  Inputs=3
  Out : Outport  OutDataType=sfix(16)  OutScaling=2^0
  wires:
  A/1 -> Mux/1
  B/1 -> Mux/2
  Mux/1 -> Fcn/1, Fcn1/1, Fcn2/1
  Fcn/1 -> Mux1/1
  Fcn1/1 -> Mux1/2
  Fcn2/1 -> Mux1/3
  Mux1/1 -> Out/1

== system starmac_system/starmac_dynamics/starmac_blade_flapping_effects/starmac_body_moments/Motor Thrust to Torques ==
  Thrusts : Inport  OutDataType=sfix(16)  OutScaling=2^0
  Demux : Demux
  Gain1 : Gain  Gain=K_torque  ParameterDataType=sfix(16)  ParameterScaling=2^0  OutDataType=sfix(16)  OutScaling=2^0
  torque 1 : Outport  OutDataType=sfix(16)  OutScaling=2^0
  torque 2 : Outport  Port=2  OutDataType=sfix(16)  OutScaling=2^0
  torque 3 : Outport  Port=3  OutDataType=sfix(16)  OutScaling=2^0
  torque 4 : Outport  Port=4  OutDataType=sfix(16)  OutScaling=2^0
  wires:
  Demux/4 -> torque 4/1
  Demux/3 -> torque 3/1
  Demux/2 -> torque 2/1
  Demux/1 -> torque 1/1
  Gain1/1 -> Demux/1
  Thrusts/1 -> Gain1/1

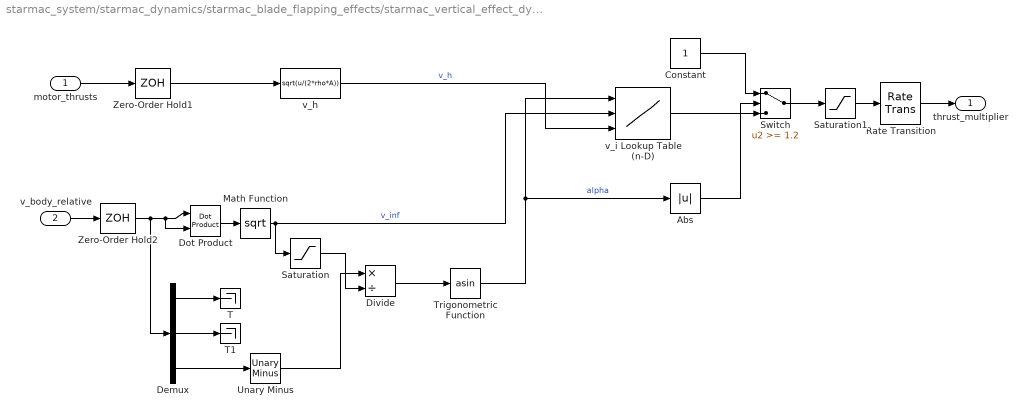
== system starmac_system/starmac_dynamics/starmac_blade_flapping_effects/starmac_vertical_effect_dynamics/starmac_motor_vertical_effect_dynamics ==
  motor_thrusts : Inport  OutDataType=sfix(16)  OutScaling=2^0
  v_body_relative : Inport  Port=2  OutDataType=sfix(16)  OutScaling=2^0
  Abs : Abs
  Constant : Constant  OutDataType=sfix(16)  OutScaling=2^0
  Demux : Demux  Outputs=3
  Divide : Product  Inputs=*/  OutDataType=sfix(16)  OutScaling=2^-10
  Dot Product : simulink/Math Operations/Dot Product  InputSameDT=on  OutDataType=sfix(16)  OutScaling=2^-10  DoSatur=off
  Math Function : Math  Operator=sqrt  OutDataType=sfix(16)  OutScaling=2^0  SaturateOnIntegerOverflow=on
  Rate Transition : RateTransition
  Saturation : Saturate  UpperLimit=500000  LowerLimit=0.0000000001
  Saturation1 : Saturate  UpperLimit=2  LowerLimit=0.5
  Switch : Switch  Threshold=1.2
  T : Terminator
  T1 : Terminator
  Trigonometric Function : Trigonometry  Operator=asin
  Unary Minus : simulink/Math Operations/Unary Minus  DoSatur=off
  Zero-Order Hold1 : ZeroOrderHold  SampleTime=tau_motor
  Zero-Order Hold2 : ZeroOrderHold  SampleTime=tau_motor
  "v_h " : Fcn  Expr=sqrt(u/(2*rho*A))
  v_i Lookup Table (n-D) : Lookup_n-D  NumberOfTableDimensions=3  BreakpointsForDimension1=Alpha  BreakpointsForDimension2=Vinf  BreakpointsForDimension3=Vh  BeginIndexSearchUsingPreviousIndexResult=on  Table=ToverTh  InterpMethod=Cubic spline  InputSameDT=on
  thrust_multiplier : Outport  OutDataType=sfix(16)  OutScaling=2^0
  wires:
  Saturation/1 -> Divide/2
  Demux/3 -> Unary Minus/1
  Unary Minus/1 -> Divide/1
  Abs/1 -> Switch/2
  Constant/1 -> Switch/1
  v_i Lookup Table (n-D)/1 -> Switch/3
  Switch/1 -> Saturation1/1
  Trigonometric Function/1 -> v_i Lookup Table (n-D)/1, Abs/1  "alpha"
  Divide/1 -> Trigonometric Function/1
  Demux/2 -> T1/1
  Demux/1 -> T/1
  Math Function/1 -> Saturation/1, v_i Lookup Table (n-D)/2  "v_inf"
  Dot Product/1 -> Math Function/1
  v_body_relative/1 -> Zero-Order Hold2/1
  motor_thrusts/1 -> Zero-Order Hold1/1
  Zero-Order Hold1/1 -> "v_h "/1
  Zero-Order Hold2/1 -> Demux/1, Dot Product/2, Dot Product/1
  Saturation1/1 -> Rate Transition/1
  "v_h "/1 -> v_i Lookup Table (n-D)/3  "v_h"
  Rate Transition/1 -> thrust_multiplier/1

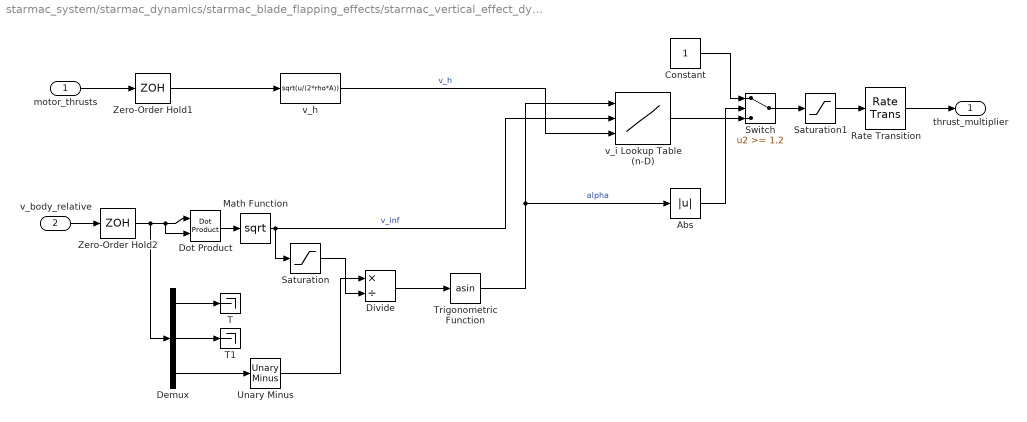
== system starmac_system/starmac_dynamics/starmac_blade_flapping_effects/starmac_vertical_effect_dynamics/starmac_motor_vertical_effect_dynamics1 ==
  motor_thrusts : Inport  OutDataType=sfix(16)  OutScaling=2^0
  v_body_relative : Inport  Port=2  OutDataType=sfix(16)  OutScaling=2^0
  Abs : Abs
  Constant : Constant  OutDataType=sfix(16)  OutScaling=2^0
  Demux : Demux  Outputs=3
  Divide : Product  Inputs=*/  OutDataType=sfix(16)  OutScaling=2^-10
  Dot Product : simulink/Math Operations/Dot Product  InputSameDT=on  OutDataType=sfix(16)  OutScaling=2^-10  DoSatur=off
  Math Function : Math  Operator=sqrt  OutDataType=sfix(16)  OutScaling=2^0  SaturateOnIntegerOverflow=on
  Rate Transition : RateTransition
  Saturation : Saturate  UpperLimit=500000  LowerLimit=0.0000000001
  Saturation1 : Saturate  UpperLimit=2  LowerLimit=0.5
  Switch : Switch  Threshold=1.2
  T : Terminator
  T1 : Terminator
  Trigonometric Function : Trigonometry  Operator=asin
  Unary Minus : simulink/Math Operations/Unary Minus  DoSatur=off
  Zero-Order Hold1 : ZeroOrderHold  SampleTime=tau_motor
  Zero-Order Hold2 : ZeroOrderHold  SampleTime=tau_motor
  "v_h " : Fcn  Expr=sqrt(u/(2*rho*A))
  v_i Lookup Table (n-D) : Lookup_n-D  NumberOfTableDimensions=3  BreakpointsForDimension1=Alpha  BreakpointsForDimension2=Vinf  BreakpointsForDimension3=Vh  BeginIndexSearchUsingPreviousIndexResult=on  Table=ToverTh  InterpMethod=Cubic spline  InputSameDT=on
  thrust_multiplier : Outport  OutDataType=sfix(16)  OutScaling=2^0
  wires:
  Saturation/1 -> Divide/2
  Demux/3 -> Unary Minus/1
  Unary Minus/1 -> Divide/1
  Abs/1 -> Switch/2
  Constant/1 -> Switch/1
  v_i Lookup Table (n-D)/1 -> Switch/3
  Switch/1 -> Saturation1/1
  Trigonometric Function/1 -> v_i Lookup Table (n-D)/1, Abs/1  "alpha"
  Divide/1 -> Trigonometric Function/1
  Demux/2 -> T1/1
  Demux/1 -> T/1
  Math Function/1 -> Saturation/1, v_i Lookup Table (n-D)/2  "v_inf"
  Dot Product/1 -> Math Function/1
  v_body_relative/1 -> Zero-Order Hold2/1
  motor_thrusts/1 -> Zero-Order Hold1/1
  Zero-Order Hold1/1 -> "v_h "/1
  Zero-Order Hold2/1 -> Demux/1, Dot Product/2, Dot Product/1
  Saturation1/1 -> Rate Transition/1
  "v_h "/1 -> v_i Lookup Table (n-D)/3  "v_h"
  Rate Transition/1 -> thrust_multiplier/1

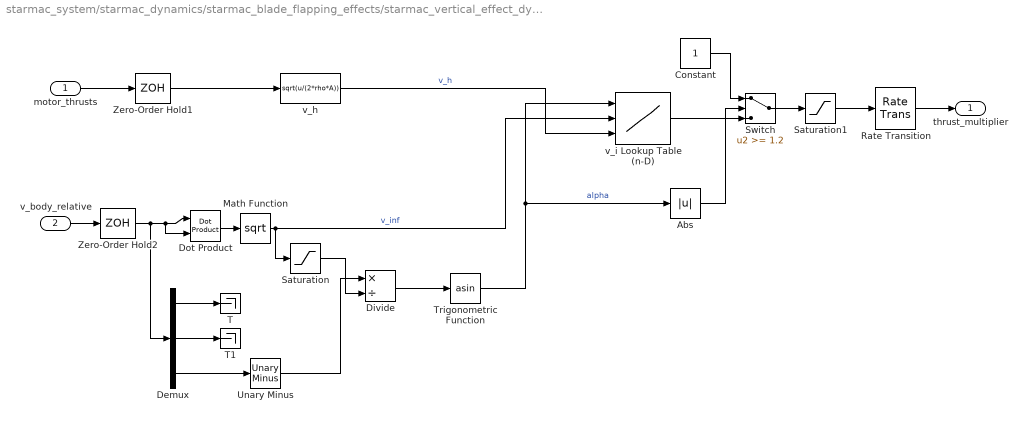
== system starmac_system/starmac_dynamics/starmac_blade_flapping_effects/starmac_vertical_effect_dynamics/starmac_motor_vertical_effect_dynamics2 ==
  motor_thrusts : Inport  OutDataType=sfix(16)  OutScaling=2^0
  v_body_relative : Inport  Port=2  OutDataType=sfix(16)  OutScaling=2^0
  Abs : Abs
  Constant : Constant  OutDataType=sfix(16)  OutScaling=2^0
  Demux : Demux  Outputs=3
  Divide : Product  Inputs=*/  OutDataType=sfix(16)  OutScaling=2^-10
  Dot Product : simulink/Math Operations/Dot Product  InputSameDT=on  OutDataType=sfix(16)  OutScaling=2^-10  DoSatur=off
  Math Function : Math  Operator=sqrt  OutDataType=sfix(16)  OutScaling=2^0  SaturateOnIntegerOverflow=on
  Rate Transition : RateTransition
  Saturation : Saturate  UpperLimit=500000  LowerLimit=0.0000000001
  Saturation1 : Saturate  UpperLimit=2  LowerLimit=0.5
  Switch : Switch  Threshold=1.2
  T : Terminator
  T1 : Terminator
  Trigonometric Function : Trigonometry  Operator=asin
  Unary Minus : simulink/Math Operations/Unary Minus  DoSatur=off
  Zero-Order Hold1 : ZeroOrderHold  SampleTime=tau_motor
  Zero-Order Hold2 : ZeroOrderHold  SampleTime=tau_motor
  "v_h " : Fcn  Expr=sqrt(u/(2*rho*A))
  v_i Lookup Table (n-D) : Lookup_n-D  NumberOfTableDimensions=3  BreakpointsForDimension1=Alpha  BreakpointsForDimension2=Vinf  BreakpointsForDimension3=Vh  BeginIndexSearchUsingPreviousIndexResult=on  Table=ToverTh  InterpMethod=Cubic spline  InputSameDT=on
  thrust_multiplier : Outport  OutDataType=sfix(16)  OutScaling=2^0
  wires:
  Saturation/1 -> Divide/2
  Demux/3 -> Unary Minus/1
  Unary Minus/1 -> Divide/1
  Abs/1 -> Switch/2
  Constant/1 -> Switch/1
  v_i Lookup Table (n-D)/1 -> Switch/3
  Switch/1 -> Saturation1/1
  Trigonometric Function/1 -> v_i Lookup Table (n-D)/1, Abs/1  "alpha"
  Divide/1 -> Trigonometric Function/1
  Demux/2 -> T1/1
  Demux/1 -> T/1
  Math Function/1 -> Saturation/1, v_i Lookup Table (n-D)/2  "v_inf"
  Dot Product/1 -> Math Function/1
  v_body_relative/1 -> Zero-Order Hold2/1
  motor_thrusts/1 -> Zero-Order Hold1/1
  Zero-Order Hold1/1 -> "v_h "/1
  Zero-Order Hold2/1 -> Demux/1, Dot Product/2, Dot Product/1
  Saturation1/1 -> Rate Transition/1
  "v_h "/1 -> v_i Lookup Table (n-D)/3  "v_h"
  Rate Transition/1 -> thrust_multiplier/1

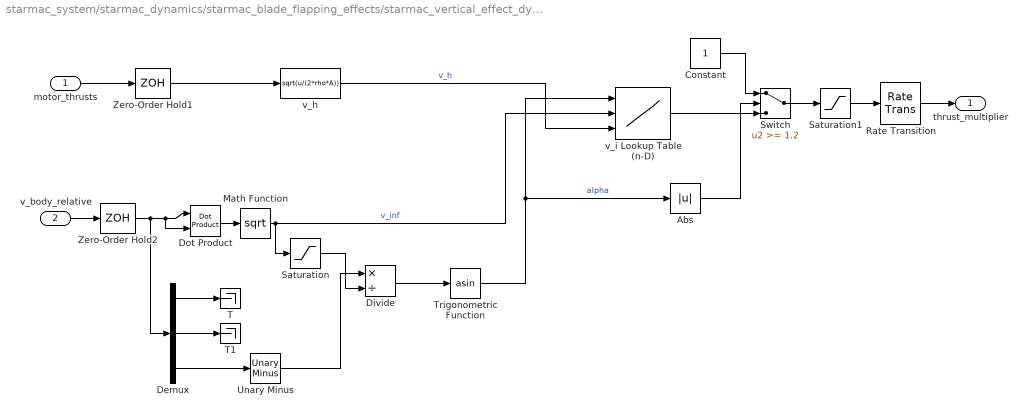
== system starmac_system/starmac_dynamics/starmac_blade_flapping_effects/starmac_vertical_effect_dynamics/starmac_motor_vertical_effect_dynamics3 ==
  motor_thrusts : Inport  OutDataType=sfix(16)  OutScaling=2^0
  v_body_relative : Inport  Port=2  OutDataType=sfix(16)  OutScaling=2^0
  Abs : Abs
  Constant : Constant  OutDataType=sfix(16)  OutScaling=2^0
  Demux : Demux  Outputs=3
  Divide : Product  Inputs=*/  OutDataType=sfix(16)  OutScaling=2^-10
  Dot Product : simulink/Math Operations/Dot Product  InputSameDT=on  OutDataType=sfix(16)  OutScaling=2^-10  DoSatur=off
  Math Function : Math  Operator=sqrt  OutDataType=sfix(16)  OutScaling=2^0  SaturateOnIntegerOverflow=on
  Rate Transition : RateTransition
  Saturation : Saturate  UpperLimit=500000  LowerLimit=0.0000000001
  Saturation1 : Saturate  UpperLimit=2  LowerLimit=0.5
  Switch : Switch  Threshold=1.2
  T : Terminator
  T1 : Terminator
  Trigonometric Function : Trigonometry  Operator=asin
  Unary Minus : simulink/Math Operations/Unary Minus  DoSatur=off
  Zero-Order Hold1 : ZeroOrderHold  SampleTime=tau_motor
  Zero-Order Hold2 : ZeroOrderHold  SampleTime=tau_motor
  "v_h " : Fcn  Expr=sqrt(u/(2*rho*A))
  v_i Lookup Table (n-D) : Lookup_n-D  NumberOfTableDimensions=3  BreakpointsForDimension1=Alpha  BreakpointsForDimension2=Vinf  BreakpointsForDimension3=Vh  BeginIndexSearchUsingPreviousIndexResult=on  Table=ToverTh  InterpMethod=Cubic spline  InputSameDT=on
  thrust_multiplier : Outport  OutDataType=sfix(16)  OutScaling=2^0
  wires:
  Saturation/1 -> Divide/2
  Demux/3 -> Unary Minus/1
  Unary Minus/1 -> Divide/1
  Abs/1 -> Switch/2
  Constant/1 -> Switch/1
  v_i Lookup Table (n-D)/1 -> Switch/3
  Switch/1 -> Saturation1/1
  Trigonometric Function/1 -> v_i Lookup Table (n-D)/1, Abs/1  "alpha"
  Divide/1 -> Trigonometric Function/1
  Demux/2 -> T1/1
  Demux/1 -> T/1
  Math Function/1 -> Saturation/1, v_i Lookup Table (n-D)/2  "v_inf"
  Dot Product/1 -> Math Function/1
  v_body_relative/1 -> Zero-Order Hold2/1
  motor_thrusts/1 -> Zero-Order Hold1/1
  Zero-Order Hold1/1 -> "v_h "/1
  Zero-Order Hold2/1 -> Demux/1, Dot Product/2, Dot Product/1
  Saturation1/1 -> Rate Transition/1
  "v_h "/1 -> v_i Lookup Table (n-D)/3  "v_h"
  Rate Transition/1 -> thrust_multiplier/1
